simulink library "FUSI_EB"  (R2023b)
settings: Solver=VariableStepAuto  StartTime=0.0  StopTime=10.0  RelTol=1e-3
settings Model: Creator=blatak  LastModifiedBy=blatak

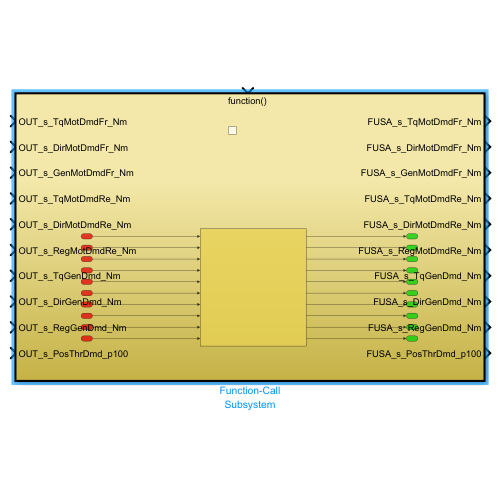
[thumbnail: Simulink's stored preview of the top-level diagram]
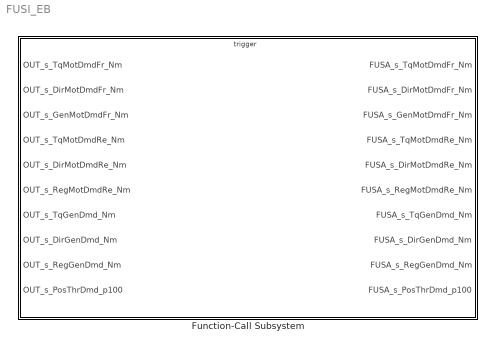
== system FUSI_EB ==
  Function-Call Subsystem : Subsystem  TreatAsAtomicUnit=on

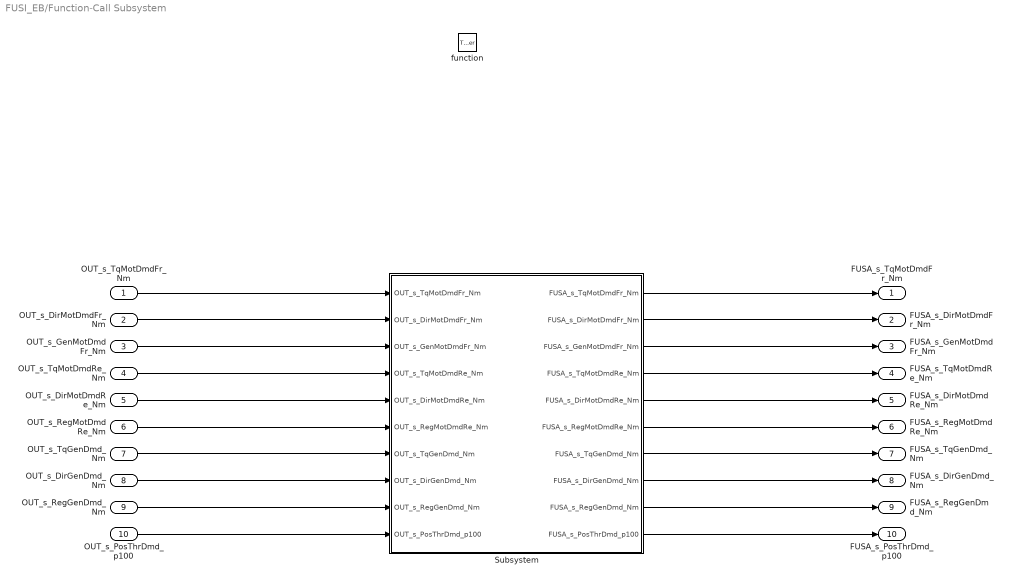
== system FUSI_EB/Function-Call Subsystem ==
  OUT_s_TqMotDmdFr_Nm : Inport
  OUT_s_DirMotDmdFr_Nm : Inport  Port=2
  OUT_s_GenMotDmdFr_Nm : Inport  Port=3
  OUT_s_TqMotDmdRe_Nm : Inport  Port=4
  OUT_s_DirMotDmdRe_Nm : Inport  Port=5
  OUT_s_RegMotDmdRe_Nm : Inport  Port=6
  OUT_s_TqGenDmd_Nm : Inport  Port=7
  OUT_s_DirGenDmd_Nm : Inport  Port=8
  OUT_s_RegGenDmd_Nm : Inport  Port=9
  OUT_s_PosThrDmd_p100 : Inport  Port=10
  function : TriggerPort  TriggerType=function-call  VariantControl=(inherit)
  Subsystem : Subsystem
  FUSA_s_TqMotDmdFr_Nm : Outport
  FUSA_s_DirMotDmdFr_Nm : Outport  Port=2
  FUSA_s_GenMotDmdFr_Nm : Outport  Port=3
  FUSA_s_TqMotDmdRe_Nm : Outport  Port=4
  FUSA_s_DirMotDmdRe_Nm : Outport  Port=5
  FUSA_s_RegMotDmdRe_Nm : Outport  Port=6
  FUSA_s_TqGenDmd_Nm : Outport  Port=7
  FUSA_s_DirGenDmd_Nm : Outport  Port=8
  FUSA_s_RegGenDmd_Nm : Outport  Port=9
  FUSA_s_PosThrDmd_p100 : Outport  Port=10
  wires:
  OUT_s_TqMotDmdFr_Nm/1 -> Subsystem/1(OUT_s_TqMotDmdFr_Nm)
  OUT_s_DirMotDmdFr_Nm/1 -> Subsystem/2(OUT_s_DirMotDmdFr_Nm)
  OUT_s_GenMotDmdFr_Nm/1 -> Subsystem/3(OUT_s_GenMotDmdFr_Nm)
  OUT_s_TqMotDmdRe_Nm/1 -> Subsystem/4(OUT_s_TqMotDmdRe_Nm)
  OUT_s_DirMotDmdRe_Nm/1 -> Subsystem/5(OUT_s_DirMotDmdRe_Nm)
  OUT_s_RegMotDmdRe_Nm/1 -> Subsystem/6(OUT_s_RegMotDmdRe_Nm)
  OUT_s_TqGenDmd_Nm/1 -> Subsystem/7(OUT_s_TqGenDmd_Nm)
  OUT_s_DirGenDmd_Nm/1 -> Subsystem/8(OUT_s_DirGenDmd_Nm)
  OUT_s_RegGenDmd_Nm/1 -> Subsystem/9(OUT_s_RegGenDmd_Nm)
  OUT_s_PosThrDmd_p100/1 -> Subsystem/10(OUT_s_PosThrDmd_p100)
  Subsystem/1(FUSA_s_TqMotDmdFr_Nm) -> FUSA_s_TqMotDmdFr_Nm/1
  Subsystem/2(FUSA_s_DirMotDmdFr_Nm) -> FUSA_s_DirMotDmdFr_Nm/1
  Subsystem/3(FUSA_s_GenMotDmdFr_Nm) -> FUSA_s_GenMotDmdFr_Nm/1
  Subsystem/4(FUSA_s_TqMotDmdRe_Nm) -> FUSA_s_TqMotDmdRe_Nm/1
  Subsystem/5(FUSA_s_DirMotDmdRe_Nm) -> FUSA_s_DirMotDmdRe_Nm/1
  Subsystem/6(FUSA_s_RegMotDmdRe_Nm) -> FUSA_s_RegMotDmdRe_Nm/1
  Subsystem/7(FUSA_s_TqGenDmd_Nm) -> FUSA_s_TqGenDmd_Nm/1
  Subsystem/8(FUSA_s_DirGenDmd_Nm) -> FUSA_s_DirGenDmd_Nm/1
  Subsystem/9(FUSA_s_RegGenDmd_Nm) -> FUSA_s_RegGenDmd_Nm/1
  Subsystem/10(FUSA_s_PosThrDmd_p100) -> FUSA_s_PosThrDmd_p100/1

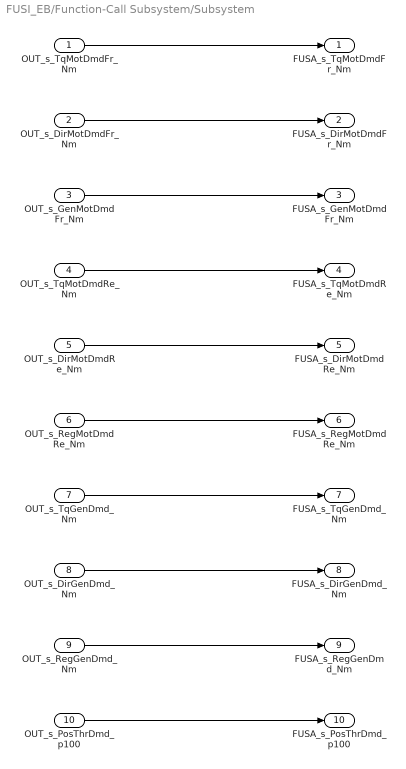
== system FUSI_EB/Function-Call Subsystem/Subsystem ==
  OUT_s_TqMotDmdFr_Nm : Inport
  OUT_s_DirMotDmdFr_Nm : Inport  Port=2
  OUT_s_GenMotDmdFr_Nm : Inport  Port=3
  OUT_s_TqMotDmdRe_Nm : Inport  Port=4
  OUT_s_DirMotDmdRe_Nm : Inport  Port=5
  OUT_s_RegMotDmdRe_Nm : Inport  Port=6
  OUT_s_TqGenDmd_Nm : Inport  Port=7
  OUT_s_DirGenDmd_Nm : Inport  Port=8
  OUT_s_RegGenDmd_Nm : Inport  Port=9
  OUT_s_PosThrDmd_p100 : Inport  Port=10
  FUSA_s_TqMotDmdFr_Nm : Outport
  FUSA_s_DirMotDmdFr_Nm : Outport  Port=2
  FUSA_s_GenMotDmdFr_Nm : Outport  Port=3
  FUSA_s_TqMotDmdRe_Nm : Outport  Port=4
  FUSA_s_DirMotDmdRe_Nm : Outport  Port=5
  FUSA_s_RegMotDmdRe_Nm : Outport  Port=6
  FUSA_s_TqGenDmd_Nm : Outport  Port=7
  FUSA_s_DirGenDmd_Nm : Outport  Port=8
  FUSA_s_RegGenDmd_Nm : Outport  Port=9
  FUSA_s_PosThrDmd_p100 : Outport  Port=10
  wires:
  OUT_s_RegMotDmdRe_Nm/1 -> FUSA_s_RegMotDmdRe_Nm/1
  OUT_s_RegGenDmd_Nm/1 -> FUSA_s_RegGenDmd_Nm/1
  OUT_s_TqMotDmdFr_Nm/1 -> FUSA_s_TqMotDmdFr_Nm/1
  OUT_s_DirMotDmdFr_Nm/1 -> FUSA_s_DirMotDmdFr_Nm/1
  OUT_s_TqMotDmdRe_Nm/1 -> FUSA_s_TqMotDmdRe_Nm/1
  OUT_s_DirMotDmdRe_Nm/1 -> FUSA_s_DirMotDmdRe_Nm/1
  OUT_s_TqGenDmd_Nm/1 -> FUSA_s_TqGenDmd_Nm/1
  OUT_s_PosThrDmd_p100/1 -> FUSA_s_PosThrDmd_p100/1
  OUT_s_DirGenDmd_Nm/1 -> FUSA_s_DirGenDmd_Nm/1
  OUT_s_GenMotDmdFr_Nm/1 -> FUSA_s_GenMotDmdFr_Nm/1
